simulink model "DC_Microgrid_Sim"  (R2023b)
settings: Solver=VariableStepDiscrete  StartTime=0.0  StopTime=72  MaxStep=1e-2  RelTol=1e-3
undefined symbols (not defined in the file or in its folder): dEgdT, EgRef, gcbh, Ion, k1, Lithium, Rsh_array5pc, sps_rtmsupport, Tref_K, Tsf, VT_ref
libraries: spsSeriesRLCBranchLib x7, spsVoltageMeasurementLib x5, SignalEditorBlockLib x2, spsCurrentMeasurementLib x2, spsDiodeLib x2, spsFirstOrderFilterLib x2, spsControlledCurrentSourceLib x2, spsPVarrayModel x2, spsBatteryLib x1, spsVariableResistorLib x1, spsBoostConverterLib x1, spsStairGeneratorLib x1
(part 1 of 9)
settings Model: SimulationMode=accelerator  Creator=andrewboland  LastModifiedBy=andrewboland

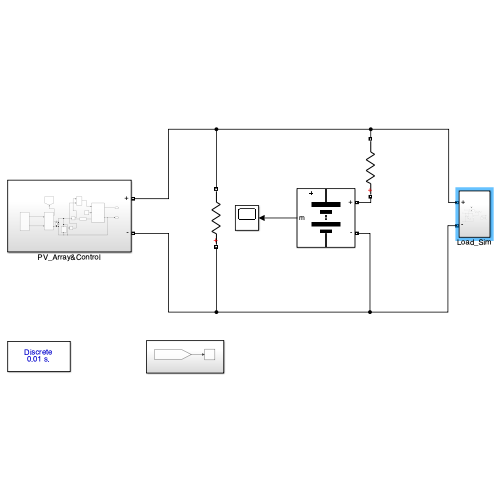
[thumbnail: Simulink's stored preview of the top-level diagram]
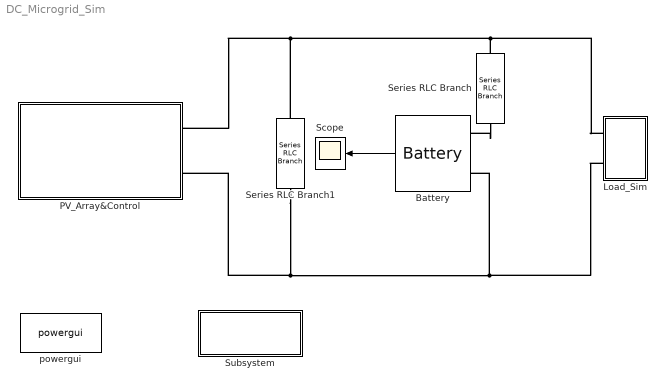
== system DC_Microgrid_Sim ==
  Battery : spsBatteryLib/Battery  BatType=Lithium-Ion  ShowTempParam=off  ThermalPreset=no  ShowAgeParam=off  NomV=400  NomQ=5  SOC=75  Batt_Tr=1  PresetModel=on  MaxQ=5  MinV=300  FullV=465.5949  Dis_rate=2.1739  R=0.8  Normal_OP=4.5217  expZone="[432.1543     0.2456522]"  current=[6.5 13 32.5]  Units=Time  Tci=20  NomT=20  T2=-30  MaxQ2=4.8  FullV2=7.1  Normal_OP2=5.655  expZone2="[6.58           1]"  Rca=0.6  ti=2000  Dp=0  Neq0=0  Tsim=1e6  Ta1=25  Qeol=5.4*0.9  Reol=0.013333*1.2  Char_age=[2.3478, 3]  Dis_age=[2.3478, 10]  N1=1500  N2=10500  N3=1000  N4=1400  Ta2=45  N5=950
  Load_Sim : Subsystem
  PV_Array&Control : Subsystem
  Scope : Scope
  Series RLC Branch : spsSeriesRLCBranchLib/Series RLC Branch  LConnTagsString=__new0  RConnTagsString=__new0  BranchType=R  Resistance=.001  Inductance=1e-3  SetiL0=off  InitialCurrent=0  Capacitance=1e-6  Setx0=off  InitialVoltage=0  Measurements=None
  Series RLC Branch1 : spsSeriesRLCBranchLib/Series RLC Branch  LConnTagsString=__new0  RConnTagsString=__new0  BranchType=R  Resistance=.001  Inductance=1e-3  SetiL0=off  InitialCurrent=0  Capacitance=1e-6  Setx0=off  InitialVoltage=0  Measurements=None
  Subsystem : Subsystem
  powergui : spspowerguiLib/powergui  Priority=1  SimulationMode=Discrete  SampleTime=1e-2  frequency=60  Iterations=50  frequencyindice=0  Pbase=100e6  ErrMax=1e-4  UnitsV=kV  UnitsW=MW  buscounter=0  FunctionMessages=off  echomessages=off  EnableUseOfTLC=off  CurrentSourceSwitches=on  DisableSnubberDevices=off  DisableRonSwitches=off  DisableVfSwitches=off  DisplayEquations=off  AutomaticDiscreteSolvers=off  SolverType=Tustin/Backward Euler (TBE)  Interpol=off  ExternalGateDelay=off  methode=off  Ts=100  x0status=blocks  SPID=on  SwTol=0  HookPort=off  NonlinearTolerance=1e-4  nMaxIteration=100  ContinueOnMaxIteration=off  RestoreLinks=warning  ResistiveCurrentMeasurement=off  Frange=[0:2:500]  Ylog=off  Xlog=on  ShowGrid=off  save=off  variable=ZData  structure=0  ZoomFFT=off  StartTime=0.0  cycles=1  DisplayStyle=1  fundamental=60  FreqAxis=off  MaxFrequency=1000  frequencyindicesteady=1  RmsSteady=1  display=off
  wires:
  Battery/1 -> Scope/1
  connections:
  Load_Sim/LConn1 -- PV_Array&Control/RConn1 -- Series RLC Branch1/RConn1 -- Series RLC Branch/RConn1
  PV_Array&Control/RConn2 -- Series RLC Branch1/LConn1 -- Load_Sim/LConn2 -- Battery/LConn2
  Series RLC Branch/LConn1 -- Battery/LConn1

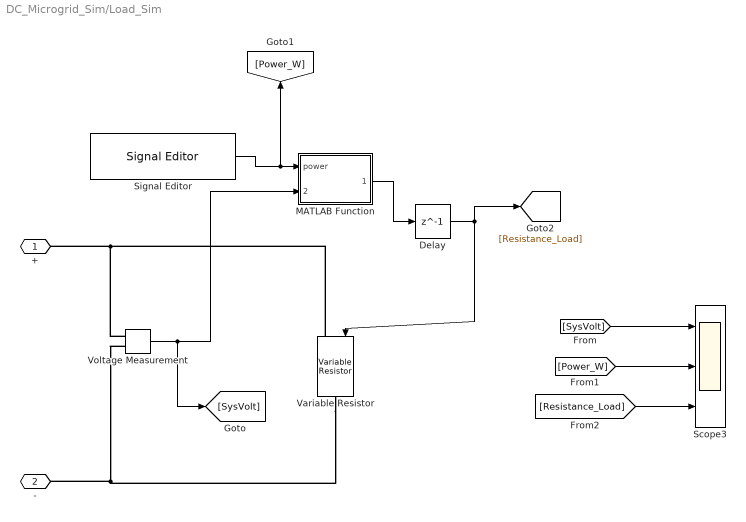
== system DC_Microgrid_Sim/Load_Sim ==
  Delay : Delay  DelayLength=1  InputProcessing=Columns as channels (frame based)
  MATLAB Function : MATLAB Function  TreatAsAtomicUnit=on
  Scope3 : Scope  NumInputPorts=3
  Signal Editor : SignalEditorBlockLib/Signal Editor  FileName=load_signal.mat  ActiveScenario=scenario  ActiveSignal=PowerConsumption  IsBus=off  OutputBusObjectStr=Bus: BusObject  SampleTime=0  Interpolate=off  ZeroCross=off  OutputAfterFinalValue=Setting to zero  Unit=inherit  PreserveSignalName=on  ApplySigPropsToAllScenarios=on  ApplySigPropsToAllSignals=off
  Variable Resistor : spsVariableResistorLib/Variable Resistor  Rabsmin=1e-8
      settings: LibrarySourceBlock=sps_lib/Passives/Variable Resistor
  Voltage Measurement : spsVoltageMeasurementLib/Voltage Measurement  PhasorSimulation=off  OutputType=Complex  PSBequivalent=0
  + : PMIOPort  Side=Left
  "-  " : PMIOPort  Port=2  Side=Left
  wires:
  Voltage Measurement/1 -> [SysVolt], MATLAB Function/2(voltage)
  MATLAB Function/1(resistance) -> Delay/1
  Delay/1 -> [Resistance_Load], Variable Resistor/1
  [SysVolt] -> Scope3/1
  Signal Editor/1 -> MATLAB Function/1(power), [Power_W]
  [Power_W] -> Scope3/2
  [Resistance_Load] -> Scope3/3
  connections:
  Variable Resistor/LConn1 -- +/RConn1 -- Voltage Measurement/LConn1
  Voltage Measurement/LConn2 -- Variable Resistor/RConn1 -- "-  "/RConn1
